simulink model "validate_stepper2"  (R2015a)
settings: Solver=ode45  StartTime=0.0  StopTime=10.0  RelTol=1e-3
undefined symbols (not defined in the file): sigbuilder_block
settings Model: CovSFcnEnable=off  Creator=hemant6043  LastModifiedBy=hemant6043
settings DebuggingCC: SolverPrmCheckMsg=warning

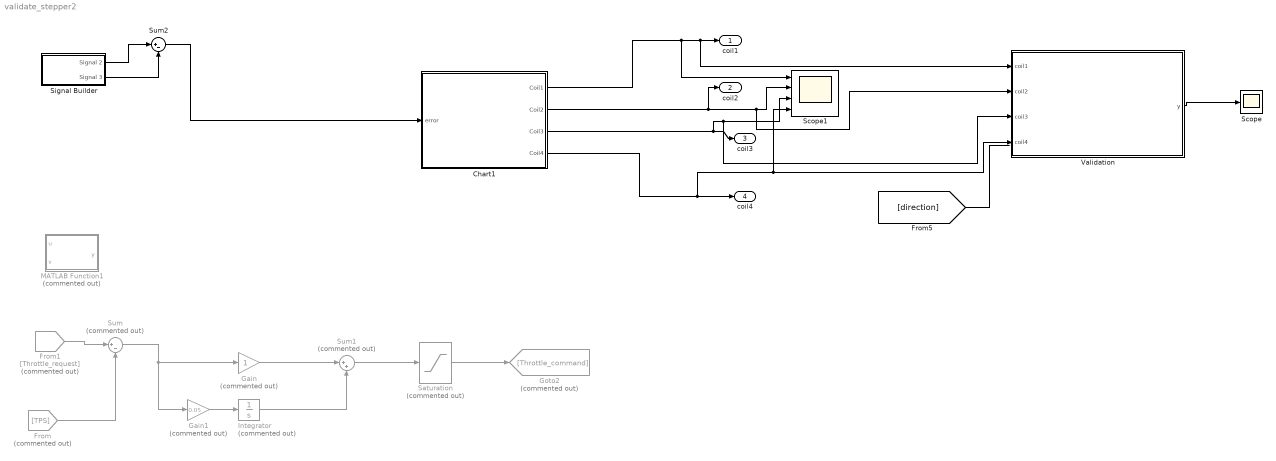
== system validate_stepper2 ==
  Chart1 : Stateflow chart  TreatAsAtomicUnit=on
  From : From  Commented=on  GotoTag=TPS
  From1 : From  Commented=on  GotoTag=Throttle_request
  Gain : Gain  Commented=on
  Gain1 : Gain  Commented=on  Gain=0.05
  Goto2 : Goto  Commented=on  GotoTag=Throttle_command
  Integrator : Integrator  Commented=on
  MATLAB Function1 : MATLAB Function  Commented=on  TreatAsAtomicUnit=on
  Saturation : Saturate  Commented=on  UpperLimit=90  LowerLimit=0
  Scope : Scope
  Scope1 : Scope  NumInputPorts=4
      settings: YMin=-5~-5~-5~-5  YMax=5~5~5~5
  Signal Builder : Subsystem  Tag=STV Subsys  LoadFcn=sigbuilder_block('load',[8.25 -228 943.5 648 ]);  StartFcn=sigbuilder_block('start');  StopFcn=sigbuilder_block('stop');  ClipboardFcn=sigbuilder_block('clipboard');  mask(Sigbuilder block){}
      mask help: Simulink:masks:SigbuilderBlock_MD
      mask init:
      | if ~strcmp(get_param(bdroot(gcbh),'SimulationStatus'),'stopped') tuvar = sigbuilder_block('maskInit'); end
      settings: CopyFcn=sigbuilder_block('copy');  DeleteFcn=sigbuilder_block('delete');  ModelCloseFcn=sigbuilder_block('modelClose');  PreSaveFcn=sigbuilder_block('preSave');  PauseFcn=sigbuilder_block('pause');  ContinueFcn=sigbuilder_block('continue');  NameChangeFcn=sigbuilder_block('namechange');  OpenFcn=sigbuilder_block('open',[451.5 -122.25 550.5 387.75 ]);  CloseFcn=sigbuilder_block('close');
      mask Display: plot(0, 0, 100, 100,[2, 2, 32, 32, 2], [68, 8, 8, 68, 68],[32, 2], [38, 38], [32, 19, 2],[53, 60, 44], [32, 17, 17, 2],[16, 16, 31, 31]);txt = getActiveGroup(gcbh);text(2, 100, txt,'verticalAlignment', 'top');
  Sum : Sum  Commented=on  Inputs=|+-
  Sum1 : Sum  Commented=on  Inputs=|++
  Sum2 : Sum  Inputs=|+-
  Validation : MATLAB Function  TreatAsAtomicUnit=on
  coil1 : Outport
  coil2 : Outport  Port=2
  coil3 : Outport  Port=3
  coil4 : Outport  Port=4
  wires:
  Chart1/1(Coil1) -> Scope1/1, Validation/1(coil1), coil1/1
  Chart1/2(Coil2) -> Validation/2(coil2), Scope1/2, coil2/1
  Chart1/3(Coil3) -> Scope1/3, Validation/3(coil3), coil3/1
  Chart1/4(Coil4) -> Validation/4(coil4), Scope1/4, coil4/1
  From1/1 -> Sum/1
  From/1 -> Sum/2
  Sum/1 -> Gain1/1, Gain/1
  Gain1/1 -> Integrator/1
  Gain/1 -> Sum1/1
  Integrator/1 -> Sum1/2
  Sum1/1 -> Saturation/1
  Saturation/1 -> Goto2/1
  [direction] -> ?
  Validation/1(y) -> Scope/1
  Signal Builder/1(Signal 2) -> Sum2/1
  Signal Builder/2(Signal 3) -> Sum2/2
  Sum2/1 -> Chart1/1(error)

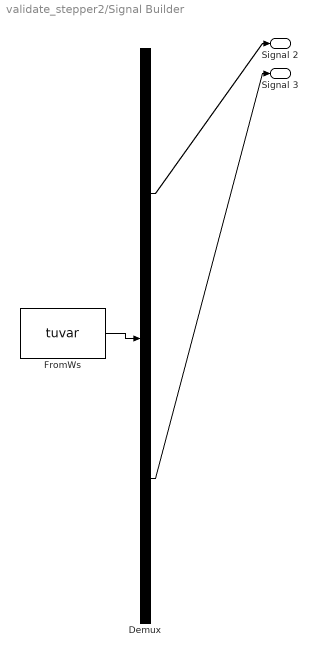
== system validate_stepper2/Signal Builder ==
  Demux : Demux  Tag=STV Demux  Outputs=2
  FromWs : FromWorkspace  Tag=STV FromWs  VariableName=tuvar  SampleTime=0
      SigBuilderData=|
      | common.afterFinalStr = 'Extrapolate'
      | common.sampleTime = 0
      | dataSet.timeRange = [0 10]
      | dataSet.name = 'Group 1'
      | sbobj.Groups.Name = 'Group 1'
      | sbobj.Groups.Signals(1).Name = 'Signal 2'
      | sbobj.Groups.Signals(1).XData = [0 1 1 2 2 3 3 4 4 5 5 6 6 7.01 7.01 8 8 9 10]
      | sbobj.Groups.Signals(1).YData = [0 0.03 12.5 12.5 25 25 37.5 37.5 50 50 35.6 35.6 75 75 60 60 100 100 100]
      | sbobj.Groups.Signals(2).Name = 'Signal 3'
      | sbobj.Groups.Signals(2).XData = [0 1 1 2 3 4 5 6 6 7.01 8 9 10]
      | sbobj.Groups.Signals(2).YData = [0 0.03 0 12.5 37.5 50 74.5 74.5 75 60 39.5 100 100]
  Signal 2 : Outport  Tag=STV Outport
  Signal 3 : Outport  Tag=STV Outport  Port=2
  wires:
  FromWs/1 -> Demux/1
  Demux/1 -> Signal 2/1
  Demux/2 -> Signal 3/1

== matlab function validate_stepper2/Validation ==
  data: coil1 input; y output; coil2 input; coil3 input; coil4 input
function y = fcn(coil1,coil2,coil3,coil4)
%#codegen
    if coil1==0&&coil2==0&&coil3==0&&coil4==0
    y=0;
    elseif coil1==1&&coil2==0&&coil3==1&&coil4==0
    y=1;
    elseif coil1==1&&coil2==0&&coil3==0&&coil4==0
    y=2;
    elseif coil1==1&&coil2==0&&coil3==0&&coil4==1
    y=3;
    elseif coil1==0&&coil2==0&&coil3==0&&coil4==1
    y=4;
    elseif coil1==0&&coil2==1&&coil3==0&&coil4==1
    y=5;
    elseif coil1==0&&coil2==1&&coil3==0&&coil4==0
    y=6;
    elseif coil1==0&&coil2==1&&coil3==1&&coil4==0
    y=7;
    elseif coil1==0&&coil2==0&&coil3==1&&coil4==0
    y=8;
    else
    y=0;
    end
 
end

== stateflow chart validate_stepper2/Chart1 ==
  state CW
    state step3
      during:
      Coil1=1
      Coil2=0
      Coil3=0
      Coil4=1
    state step2
      during:
      Coil1=1
      Coil2=0
      Coil3=0
      Coil4=0
    state Step0
      during:
      Coil1=0
      Coil2=0
      Coil3=0
      Coil4=0
    state step1
      during:
      Coil1=1
      Coil2=0
      Coil3=1
      Coil4=0
    state step6
      during:
      Coil1=0
      Coil2=1
      Coil3=0
      Coil4=0
    state step5
      during:
      Coil1=0
      Coil2=1
      Coil3=0
      Coil4=1
    state step4
      during:
      Coil1=0
      Coil2=0
      Coil3=0
      Coil4=1
    state step8
      during:
      Coil1=0
      Coil2=0
      Coil3=1
      Coil4=0
    state step7
      during:
      Coil1=0
      Coil2=1
      Coil3=1
      Coil4=0
    (default) -> Step0
    step2 -> step3 [order 2] : [error>=12.5]
    step1 -> step2 [order 1] : [error>=12.5]
    Step0 -> step1 : [error>=12.5]
    step3 -> step2 [order 1] : [error<-12.5]
    step2 -> step1 [order 1] : [error<-12.5]
    step1 -> Step0 [order 2] : [error<-12.5]
    step3 -> step4 [order 2] : [error>=12.5]
    step4 -> step3 [order 1] : [error<-12.5]
    step4 -> step5 [order 2] : [error>=12.5]
    step5 -> step6 [order 2] : [error>=12.5]
    step6 -> step5 [order 1] : [error<-12.5]
    step5 -> step4 [order 1] : [error<-12.5]
    step6 -> step7 [order 2] : [error>=12.5]
    step7 -> step6 [order 1] : [error<-12.5]
    step7 -> step8 [order 2] : [error>=12.5]
    step8 -> step7 : [error<-12.5]
  data: Coil1 output; Coil2 output; Coil3 output; Coil4 output; error input

== matlab function validate_stepper2/MATLAB Function1 ==
  data: u input; y output; v input
function y = fcn(u,v)
%#codegen
Diff=u-v;
if abs(Diff)>=1
    if Diff>0
        y=1;
    elseif Diff<0
        y=0;
    else
        y=-1;
    end
else 
    y=-1;
end
end
